simulink model "DCM_17_Parrllel_Pairs_18Ms"  (R2019b)
settings: Solver=VariableStepAuto  StartTime=0.0  StopTime=20  RelTol=1e-3
model workspace (MAT data in the model file):
  Laf = 0.00735
  Laf_2 = 0.00844
  Rarm = 0.0096
  angular_vel = 145
  angular_vel_1 = 175.405
  angular_vel_10 = 168.703
  angular_vel_11 = 168.598
  angular_vel_12 = 167.865
  angular_vel_13 = 167.132
  angular_vel_14 = 166.923
  angular_vel_15 = 165.666
  angular_vel_16 = 164.41
  angular_vel_2 = 173.625
  angular_vel_3 = 172.787
  angular_vel_4 = 170.902
  angular_vel_5 = 170.902
  angular_vel_6 = 169.96
  angular_vel_7 = 169.855
  angular_vel_8 = 169.122
libraries: powerlib x74, simulink x1
settings Model: OrderedModelArguments=off  Creator=Sy2  LastModifiedBy=Sy2
settings SolverCC: ZeroCrossAlgorithm=Adaptive
settings DebuggingCC: IgnoredZcDiagnostic=none

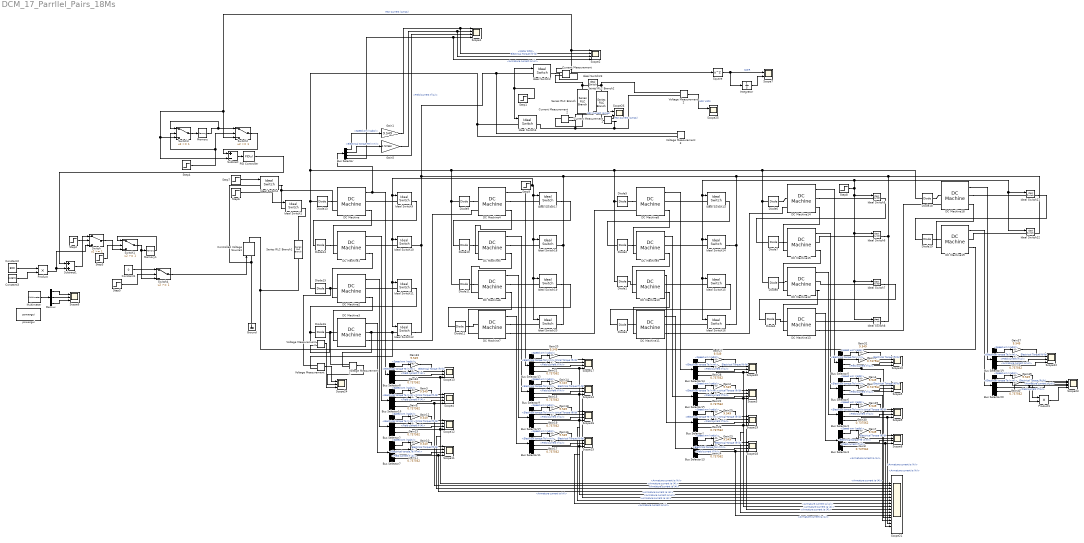
== system DCM_17_Parrllel_Pairs_18Ms ==
  Bus Selector{,1..16,19..20} (19 alike) : BusSelector  OutputSignals=Speed wm (rad/s),Electrical torque Te (n m),Field current if (A),Armature current ia (A)
  Constant1 : Constant  Value=0
  Constant2 : Constant  Value=800
  Constant3 : Constant  Value=0.0972
  Controlled Voltage Source1 : powerlib/Electrical Sources/Controlled Voltage Source  Initialize=on  Source_Type=DC  Amplitude=0  Phase=0  Frequency=0  Measurements=Voltage
      settings: SourceProductName=Simscape Electrical
  Current Measurement : powerlib/Measurements/Current Measurement  PhasorSimulation=off  OutputType=Complex  PSBequivalent=0
      settings: SourceProductName=Simscape Electrical
  Current Measurement1 : powerlib/Measurements/Current Measurement  PhasorSimulation=off  OutputType=Complex  PSBequivalent=0
      settings: SourceProductName=Simscape Electrical
  Current Measurement2 : powerlib/Measurements/Current Measurement  PhasorSimulation=off  OutputType=Complex  PSBequivalent=0
      settings: SourceProductName=Simscape Electrical
  DC Machine{,1..15,18..19} (18 alike) : powerlib/Machines/DC Machine  PresetModel=No  MechanicalLoad=Torque TL  FieldType=Wound  ShowDetailedParameters=on  MeasurementBus=off  RLa="[Rarm  0.002]"  RLf=[0.0054 0.0125]  Laf=Laf  MachineConstant=Torque constant (N.m/A)  Ke=1.8  Kt=1.8  J=137  Bm=0  Tf=0  w0=angular_vel  Ifinit=0  TsPowergui=0  TsBlock=-1
      settings: SourceProductName=Simscape Electrical
  Demux : Demux  Outputs=3
  Diode{1..2,4,6..12,14,18..19} (13 alike) : powerlib/Power Electronics/Diode  Ron=0.001  Lon=0  Vf=0.8  IC=0  UseSnubber=0  Rs=500000  Cs=250e-9  Measurements=off
      settings: SourceProductName=Simscape Electrical
  Diode13 : powerlib/Power Electronics/Diode  Ron=0.0000001  Lon=0  Vf=0.8  IC=0  UseSnubber=0  Rs=500000  Cs=250e-9  Measurements=off
      settings: SourceProductName=Simscape Electrical
  Diode15 : powerlib/Power Electronics/Diode  Ron=0.000000000001  Lon=0  Vf=0.8  IC=0  UseSnubber=0  Rs=inf  Cs=0  Measurements=off
      settings: SourceProductName=Simscape Electrical
  Diode16 : powerlib/Power Electronics/Diode  Ron=0.000000001  Lon=0  Vf=0.8  IC=0  UseSnubber=0  Rs=inf  Cs=0  Measurements=off
      settings: SourceProductName=Simscape Electrical
  Diode3 : powerlib/Power Electronics/Diode  Ron=0.00001  Lon=0  Vf=0.8  IC=0  UseSnubber=0  Rs=500000  Cs=250e-9  Measurements=off
      settings: SourceProductName=Simscape Electrical
  Diode5 : powerlib/Power Electronics/Diode  Ron=0.000001  Lon=0  Vf=0.8  IC=0  UseSnubber=0  Rs=500000  Cs=250e-9  Measurements=off
      settings: SourceProductName=Simscape Electrical
  Gain{1..4,7,10,12,14,16,18,20,23,25,27,29,31,33,37,39} (19 alike) : Gain  Gain=9.549
  Gain{5..6,8..9,11,13,15,17,19,21..22,24,26,28,30,32,34,38,40} (19 alike) : Gain  Gain=0.737562
  Ground : powerlib/Elements/Ground  LConnTagsString=a
      settings: SourceProductName=Simscape Electrical
  Ideal Switch{1..3,5..23} (22 alike) : powerlib/Power Electronics/Ideal Switch  Ron=0  Lon=0  IC=0  Rs=inf  Cs=0  Measurements=on
      settings: SourceProductName=Simscape Electrical
  Ideal Switch4 : powerlib/Power Electronics/Ideal Switch  Ron=0  Lon=0  IC=1  Rs=inf  Cs=0  Measurements=on
      settings: SourceProductName=Simscape Electrical
  Integrator : Integrator  ZeroCross=off
  Memory : Memory
  Memory1 : Memory
  Multimeter : powerlib/Measurements/Multimeter  PhasorSimulation=off  OutputType=Complex  sel=[2 3 1]  L=3  Gain=[1 1 1]  yselected={'Usrc: Controlled Voltage Source1','Ib: Series RLC Branch1','Ub: Series RLC Branch1'};  PSBOutputType=1  PSBequivalent=0  AxesSetting=[0,0.1,-100,100]  Display=0  SavedBlockNames=-11
      settings: SourceProductName=Simscape Electrical
  PID Controller : simulink/Continuous/PID Controller  Controller=PID  Form=Parallel  TimeDomain=Continuous-time  SampleTime=-1  IntegratorMethod=Forward Euler  FilterMethod=Forward Euler  ControllerParametersSource=internal  P=10  I=7  D=1  UseFilter=on  N=100  TunerSelectOption=Transfer Function Based (PID Tuner App)  InitialConditionSource=internal  InitialConditionForIntegrator=0  InitialConditionForFilter=0  DifferentiatorICPrevScaledInput=0  ExternalReset=none  TrackingMode=off  Kt=1  LimitOutput=off  UpperSaturationLimit=inf  LowerSaturationLimit=-inf  LinearizeAsGain=on  AntiWindupMode=none  Kb=1  POutMin=[]  POutMax=[]  IOutMin=[]  IOutMax=[]  DOutMin=[]  DOutMax=[]  NOutMin=[]  NOutMax=[]  SumOutMin=[]  SumOutMax=[]  SaturationOutMin=[]  SaturationOutMax=[]  PParamMin=[]  PParamMax=[]  IParamMin=[]  IParamMax=[]  DParamMin=[]  DParamMax=[]  NParamMin=[]  NParamMax=[]  KbParamMin=[]  KbParamMax=[]  KtParamMin=[]  KtParamMax=[]  KbOutMin=[]  KbOutMax=[]  KtOutMin=[]  KtOutMax=[]  IntegratorOutMin=[]  IntegratorOutMax=[]  FilterOutMin=[]  FilterOutMax=[]  SumI1OutMin=[]  SumI1OutMax=[]  SumI2OutMin=[]  SumI2OutMax=[]  SumI3OutMin=[]  SumI3OutMax=[]  SumI4OutMin=[]  SumI4OutMax=[]  SumDOutMin=[]  SumDOutMax=[]  DifferentiatorOutMin=[]  DifferentiatorOutMax=[]  FilterDiffOutCoefMin=[]  FilterDiffOutCoefMax=[]  ReciprocalOutMin=[]  ReciprocalOutMax=[]  SumDenOutMin=[]  SumDenOutMax=[]  SumNumOutMin=[]  SumNumOutMax=[]  DivideOutMin=[]  DivideOutMax=[]  IntegratorContinuousStateAttributes=''  IntegratorStateMustResolveToSignalObject=off  IntegratorRTWStateStorageClass=Auto  FilterContinuousStateAttributes=''  FilterStateMustResolveToSignalObject=off  FilterRTWStateStorageClass=Auto  ParallelPVariant=InternalParameters  IdealPVariant=Disabled  IVariant=InternalParameters  DVariant=InternalParameters  IntegratorVariant=Continuous  SatVariant=Disabled  AWVariant=Passthrough  PCopyVariant=Disabled  TRVariant=Disabled  FdbkBlocksVariant=Forward  IdealPFdbkVariant=Disabled  SatFdbkVariant=Disabled  DerivativeFilterVariant=ContFilter  NVariant=InternalParameters  NCopyVariant=Disabled  FilterICVariant=InternalICsFilter  IntegratorICVariant=InternalICs  ExternalResetVariant=Disabled  TRSumVariant=Passthrough  SumFdbkVariant=Disabled  SumVariant=Sum_PID
  Product : Product
  Product1 : Product
  Scope{1..5,8..20,22} (19 alike) : Scope  NumInputPorts=4
  Scope21 : Scope  NumInputPorts=16
  Scope23 : Scope  NumInputPorts=5
  Scope24 : Scope  NumInputPorts=3
  Scope25 : Scope  NumInputPorts=2
  Scope26 : Scope  NumInputPorts=2
  Scope6 : Scope  NumInputPorts=3
  Scope7 : Scope  NumInputPorts=2
  Series RLC Branch : powerlib/Elements/Series RLC Branch  LConnTagsString=__new0  RConnTagsString=__new0  BranchType=RL  Resistance=0.09  Inductance=0.02  SetiL0=off  InitialCurrent=0  Capacitance=1e-6  Setx0=off  InitialVoltage=0  Measurements=None
      settings: SourceProductName=Simscape Electrical
  Series RLC Branch1 : powerlib/Elements/Series RLC Branch  Description=Field Dump Resistor  LConnTagsString=__new0  RConnTagsString=__new0  BranchType=R  Resistance=5  Inductance=1e-3  SetiL0=off  InitialCurrent=0  Capacitance=1e-6  Setx0=off  InitialVoltage=0  Measurements=Branch voltage and current
      settings: AttributesFormatString=%<Description>  SourceProductName=Simscape Electrical
  Series RLC Branch2 : powerlib/Elements/Series RLC Branch  LConnTagsString=__new0  RConnTagsString=__new0  BranchType=RL  Resistance=0.90  Inductance=0.015  SetiL0=off  InitialCurrent=0  Capacitance=1e-6  Setx0=off  InitialVoltage=0  Measurements=None
      settings: SourceProductName=Simscape Electrical
  Square : Math  Operator=square  RndMeth=Zero  SaturateOnIntegerOverflow=on
  Step1 : Step  Time=12  SampleTime=0  VectorParams1D=off
  Step{2..3,5..6} (4 alike) : Step  Time=13  SampleTime=0  VectorParams1D=off  ZeroCross=off
  Step4 : Step  Time=12.72  SampleTime=0  VectorParams1D=off  ZeroCross=off
  Step7 : Step  Time=13  Before=1  After=0  SampleTime=0  VectorParams1D=off  ZeroCross=off
  Step8 : Step  Time=12  SampleTime=0  VectorParams1D=off
  Step9 : Step  Time=12  SampleTime=0  VectorParams1D=off
  Subtract : Sum  Inputs=+-
  Subtract1 : Sum
  Switch{,1..4} (5 alike) : Switch  Threshold=1  ZeroCross=off
  Voltage Measurement{,1..4} (5 alike) : powerlib/Measurements/Voltage Measurement  PhasorSimulation=off  OutputType=Complex  PSBequivalent=0
      settings: SourceProductName=Simscape Electrical
  powergui : powerlib/powergui  Priority=1  SimulationMode=Continuous  SampleTime=50e-6  frequency=60  Iterations=50  frequencyindice=0  Pbase=100e6  ErrMax=1e-4  UnitsV=kV  UnitsW=MW  buscounter=0  FunctionMessages=off  echomessages=off  EnableUseOfTLC=off  CurrentSourceSwitches=off  DisableSnubberDevices=off  DisableRonSwitches=off  DisableVfSwitches=off  DisplayEquations=off  AutomaticDiscreteSolvers=off  SolverType=Tustin/Backward Euler (TBE)  Interpol=off  ExternalGateDelay=off  methode=off  Ts=100  x0status=blocks  SPID=on  SwTol=0  HookPort=off  NonlinearTolerance=1e-4  nMaxIteration=100  ContinueOnMaxIteration=off  RestoreLinks=warning  ResistiveCurrentMeasurement=off  Frange=[0:2:500]  Ylog=off  Xlog=on  ShowGrid=off  save=off  variable=ZData  structure=0  ZoomFFT=off  StartTime=0.0  cycles=1  DisplayStyle=1  fundamental=60  FreqAxis=off  MaxFrequency=1000  frequencyindicesteady=1  RmsSteady=1  display=off
      settings: SourceProductName=Simscape Electrical
  wires:
  Bus Selector/1 -> Gain1/1  "<Speed wm (rad/s)>"
  Bus Selector/3 -> Scope1/3  "<Field current if (A)>"
  Bus Selector/4 -> Scope2/4, Scope1/4  "<Armature current ia (A)>"
  Gain1/1 -> Scope1/1, Scope2/2  "<Motor RPM>"
  Step1/1 -> Ideal Switch2/1, Ideal Switch3/1
  Step2/1 -> Switch/2
  Current Measurement/1 -> Square/1, Switch2/3, Switch3/3, Subtract/2, Scope2/1  "HSX Current (Amps)"
  Memory/1 -> Switch3/1, Switch2/1
  Subtract/1 -> PID Controller/1
  PID Controller/1 -> Subtract1/1
  Constant2/1 -> Product/1
  Subtract1/1 -> Switch/1
  Step3/1 -> Switch1/2
  Switch2/1 -> Subtract/1
  Step4/1 -> Switch2/2, Switch3/2
  Switch3/1 -> Memory/1
  Bus Selector/2 -> Gain5/1  "<Electrical torque Te (n m)>"
  Gain5/1 -> Scope2/3, Scope1/2  "Electrical Torque (ft-lb)"
  Square/1 -> Scope7/1, Integrator/1  "Isq*R"
  Integrator/1 -> Scope7/2
  Switch4/1 -> Controlled Voltage Source1/1
  Step5/1 -> Switch4/2
  Constant1/1 -> Switch4/1
  Step6/1 -> Ideal Switch1/1
  Step7/1 -> Ideal Switch4/1
  Constant3/1 -> Product/2
  Product/1 -> Subtract1/2, Switch/3
  Switch/1 -> Switch1/3
  Switch1/1 -> Switch4/3, Memory1/1
  Memory1/1 -> Switch1/1
  Demux/2 -> Scope6/2
  Multimeter/1 -> Demux/1
  Demux/1 -> Scope6/1
  Demux/3 -> Scope6/3
  Step9/1 -> Ideal Switch12/1, Ideal Switch11/1, Ideal Switch10/1, Ideal Switch9/1, Ideal Switch17/1, Ideal Switch19/1, Ideal Switch20/1, Ideal Switch18/1
  Bus Selector9/2 -> Gain15/1  "<Electrical torque Te (n m)>"
  Bus Selector9/3 -> Scope14/3  "<Field current if (A)>"
  DC Machine5/1 -> Bus Selector9/1
  Bus Selector10/3 -> Scope16/3  "<Field current if (A)>"
  Gain15/1 -> Scope14/2  "Electrical Torque (ft-lb)"
  Bus Selector9/4 -> Scope21/6, Scope14/4  "<Armature current ia (A)>"
  Gain14/1 -> Scope14/1
  Bus Selector9/1 -> Gain14/1  "<Speed wm (rad/s)>"
  Bus Selector10/1 -> Gain18/1  "<Speed wm (rad/s)>"
  DC Machine7/1 -> Bus Selector11/1
  Gain19/1 -> Scope16/2  "Electrical Torque (ft-lb)"
  Bus Selector11/4 -> Scope21/8, Scope15/4  "<Armature current ia (A)>"
  Bus Selector10/4 -> Scope21/7, Scope16/4  "<Armature current ia (A)>"
  Gain18/1 -> Scope16/1
  DC Machine6/1 -> Bus Selector10/1
  Gain16/1 -> Scope15/1
  Bus Selector11/1 -> Gain16/1  "<Speed wm (rad/s)>"
  Bus Selector11/3 -> Scope15/3  "<Field current if (A)>"
  Bus Selector11/2 -> Gain17/1  "<Electrical torque Te (n m)>"
  Gain17/1 -> Scope15/2  "Electrical Torque (ft-lb)"
  Bus Selector10/2 -> Gain19/1  "<Electrical torque Te (n m)>"
  Gain20/1 -> Scope17/1
  Bus Selector12/4 -> Scope21/5, Scope17/4  "<Armature current ia (A)>"
  Gain21/1 -> Scope17/2  "Electrical Torque (ft-lb)"
  Bus Selector12/1 -> Gain20/1  "<Speed wm (rad/s)>"
  Bus Selector12/3 -> Scope17/3  "<Field current if (A)>"
  Bus Selector12/2 -> Gain21/1  "<Electrical torque Te (n m)>"
  DC Machine4/1 -> Bus Selector12/1
  DC Machine10/1 -> Bus Selector1/1
  Bus Selector14/3 -> Scope20/3  "<Field current if (A)>"
  Bus Selector14/2 -> Gain28/1  "<Electrical torque Te (n m)>"
  Gain28/1 -> Scope20/2  "Electrical Torque (ft-lb)"
  Bus Selector14/1 -> Gain27/1  "<Speed wm (rad/s)>"
  Gain27/1 -> Scope20/1
  Bus Selector14/4 -> Scope21/9, Scope20/4  "<Armature current ia (A)>"
  DC Machine8/1 -> Bus Selector14/1
  Bus Selector13/1 -> Gain23/1  "<Speed wm (rad/s)>"
  Gain24/1 -> Scope18/2  "Electrical Torque (ft-lb)"
  Gain23/1 -> Scope18/1
  Bus Selector13/2 -> Gain24/1  "<Electrical torque Te (n m)>"
  Gain25/1 -> Scope19/1
  DC Machine9/1 -> Bus Selector15/1
  Gain26/1 -> Scope19/2  "Electrical Torque (ft-lb)"
  Bus Selector13/3 -> Scope18/3  "<Field current if (A)>"
  Bus Selector1/1 -> Gain25/1  "<Speed wm (rad/s)>"
  Gain2/1 -> Scope3/1
  Bus Selector1/3 -> Scope19/3  "<Field current if (A)>"
  Bus Selector1/4 -> Scope21/11, Scope19/4  "<Armature current ia (A)>"
  Bus Selector15/4 -> Scope21/10, Scope3/4  "<Armature current ia (A)>"
  Gain22/1 -> Scope3/2  "Electrical Torque (ft-lb)"
  DC Machine11/1 -> Bus Selector13/1
  Bus Selector15/1 -> Gain2/1  "<Speed wm (rad/s)>"
  Bus Selector1/2 -> Gain26/1  "<Electrical torque Te (n m)>"
  Bus Selector15/3 -> Scope3/3  "<Field current if (A)>"
  Bus Selector15/2 -> Gain22/1  "<Electrical torque Te (n m)>"
  DC Machine12/1 -> Bus Selector3/1
  Bus Selector5/3 -> Scope10/3  "<Field current if (A)>"
  Bus Selector5/2 -> Gain32/1  "<Electrical torque Te (n m)>"
  Gain32/1 -> Scope10/2  "Electrical Torque (ft-lb)"
  Bus Selector5/1 -> Gain31/1  "<Speed wm (rad/s)>"
  Gain31/1 -> Scope10/1
  Bus Selector5/4 -> Scope21/13, Scope10/4  "<Armature current ia (A)>"
  DC Machine14/1 -> Bus Selector5/1
  Bus Selector4/1 -> Gain7/1  "<Speed wm (rad/s)>"
  Gain8/1 -> Scope8/2  "Electrical Torque (ft-lb)"
  Gain7/1 -> Scope8/1
  Bus Selector4/2 -> Gain8/1  "<Electrical torque Te (n m)>"
  Gain29/1 -> Scope9/1
  DC Machine15/1 -> Bus Selector6/1
  Gain30/1 -> Scope9/2  "Electrical Torque (ft-lb)"
  Bus Selector4/3 -> Scope8/3  "<Field current if (A)>"
  Bus Selector4/4 -> Scope8/4, Scope21/16  "<Armature current ia (A)>"
  Bus Selector3/1 -> Gain29/1  "<Speed wm (rad/s)>"
  Gain4/1 -> Scope5/1
  Bus Selector3/3 -> Scope9/3  "<Field current if (A)>"
  Bus Selector3/4 -> Scope21/15, Scope9/4  "<Armature current ia (A)>"
  Bus Selector6/4 -> Scope21/14, Scope5/4  "<Armature current ia (A)>"
  Gain6/1 -> Scope5/2  "Electrical Torque (ft-lb)"
  DC Machine13/1 -> Bus Selector4/1
  Bus Selector6/1 -> Gain4/1  "<Speed wm (rad/s)>"
  Bus Selector3/2 -> Gain30/1  "<Electrical torque Te (n m)>"
  Bus Selector6/3 -> Scope5/3  "<Field current if (A)>"
  Bus Selector6/2 -> Gain6/1  "<Electrical torque Te (n m)>"
  DC Machine2/1 -> Bus Selector2/1
  Bus Selector8/3 -> Scope13/3  "<Field current if (A)>"
  Bus Selector8/2 -> Gain34/1  "<Electrical torque Te (n m)>"
  Gain34/1 -> Scope13/2  "Electrical Torque (ft-lb)"
  Bus Selector8/1 -> Gain33/1  "<Speed wm (rad/s)>"
  Gain33/1 -> Scope13/1
  Bus Selector8/4 -> Scope21/1, Scope13/4  "<Armature current ia (A)>"
  DC Machine/1 -> Bus Selector8/1, Bus Selector/1
  Bus Selector7/1 -> Gain10/1  "<Speed wm (rad/s)>"
  Gain11/1 -> Scope11/2  "Electrical Torque (ft-lb)"
  Gain10/1 -> Scope11/1
  Bus Selector7/2 -> Gain11/1  "<Electrical torque Te (n m)>"
  Gain12/1 -> Scope12/1
  DC Machine1/1 -> Bus Selector16/1
  Gain13/1 -> Scope12/2  "Electrical Torque (ft-lb)"
  Bus Selector7/3 -> Scope11/3  "<Field current if (A)>"
  Bus Selector7/4 -> Scope11/4, Scope21/4  "<Armature current ia (A)>"
  Bus Selector2/1 -> Gain12/1  "<Speed wm (rad/s)>"
  Gain3/1 -> Scope4/1
  Bus Selector2/3 -> Scope12/3  "<Field current if (A)>"
  Bus Selector2/4 -> Scope21/3, Scope12/4  "<Armature current ia (A)>"
  Gain9/1 -> Scope4/2  "Electrical Torque (ft-lb)"
  DC Machine3/1 -> Bus Selector7/1
  Bus Selector16/1 -> Gain3/1  "<Speed wm (rad/s)>"
  Bus Selector2/2 -> Gain13/1  "<Electrical torque Te (n m)>"
  Bus Selector16/3 -> Scope4/3  "<Field current if (A)>"
  Bus Selector16/2 -> Gain9/1  "<Electrical torque Te (n m)>"
  Bus Selector16/4 -> Scope21/2, Scope4/4  "<Armature current ia (A)>"
  Bus Selector13/4 -> Scope21/12, Scope18/4  "<Armature current ia (A)>"
  Bus Selector19/3 -> Scope22/3  "<Field current if (A)>"
  Gain40/1 -> Scope23/2  "Electrical Torque (ft-lb)"
  Bus Selector20/1 -> Gain39/1  "<Speed wm (rad/s)>"
  Bus Selector19/1 -> Gain37/1  "<Speed wm (rad/s)>"
  Bus Selector20/3 -> Scope23/3  "<Field current if (A)>"
  Bus Selector19/2 -> Gain38/1  "<Electrical torque Te (n m)>"
  Bus Selector19/4 -> Scope22/4  "<Armature current ia (A)>"
  DC Machine18/1 -> Bus Selector19/1
  Gain37/1 -> Scope22/1
  Step8/1 -> Ideal Switch22/1, Ideal Switch21/1, Ideal Switch15/1, Ideal Switch16/1, Ideal Switch14/1, Ideal Switch13/1, Ideal Switch8/1, Ideal Switch7/1, Ideal Switch6/1, Ideal Switch5/1
  DC Machine19/1 -> Bus Selector20/1
  Bus Selector20/4 -> Product1/2, Scope23/4  "<Armature current ia (A)>"
  Gain38/1 -> Scope22/2  "Electrical Torque (ft-lb)"
  Bus Selector20/2 -> Gain40/1  "<Electrical torque Te (n m)>"
  Gain39/1 -> Product1/1, Scope23/1
  Voltage Measurement/1 -> Scope24/1
  Voltage Measurement1/1 -> Scope24/2
  Voltage Measurement2/1 -> Scope25/1  "HSX Volts"
  Voltage Measurement4/1 -> Scope24/3
  Current Measurement2/1 -> Scope26/1  "HSX Current (Amps)"
  Current Measurement1/1 -> Scope26/2  "HSX Current (Amps)"
  Product1/1 -> Scope23/5
  connections:
  Voltage Measurement2/LConn2 -- Current Measurement1/RConn1 -- Ideal Switch3/RConn1 -- Current Measurement2/RConn1
  Ideal Switch12/RConn1 -- Ideal Switch20/RConn1 -- Ideal Switch18/RConn1 -- Ideal Switch8/RConn1 -- Ideal Switch6/RConn1 -- Ideal Switch22/RConn1 -- Ideal Switch16/RConn1 -- Ideal Switch14/RConn1 -- Ideal Switch2/LConn1 -- Voltage Measurement3/LConn1 -- Ideal Switch10/RConn1
  DC Machine/RConn2 -- DC Machine1/LConn2
  DC Machine1/RConn2 -- DC Machine2/LConn2
  DC Machine2/RConn2 -- DC Machine3/LConn2
  DC Machine3/RConn2 -- DC Machine4/LConn2
  DC Machine4/RConn2 -- DC Machine5/LConn2
  DC Machine5/RConn2 -- DC Machine6/LConn2
  DC Machine6/RConn2 -- DC Machine7/LConn2
  DC Machine7/RConn2 -- DC Machine8/LConn2
  DC Machine8/RConn2 -- DC Machine9/LConn2
  DC Machine9/RConn2 -- DC Machine10/LConn2
  DC Machine10/RConn2 -- DC Machine11/LConn2
  DC Machine11/RConn2 -- DC Machine14/LConn2
  DC Machine14/RConn2 -- DC Machine15/LConn2
  DC Machine15/RConn2 -- DC Machine12/LConn2
  DC Machine12/RConn2 -- DC Machine13/LConn2
  DC Machine/LConn2 -- Ideal Switch4/RConn1 -- Ideal Switch1/LConn1
  Ideal Switch1/RConn1 -- Series RLC Branch1/LConn1
  Ideal Switch9/LConn1 -- DC Machine/RConn1
  Ideal Switch10/LConn1 -- DC Machine1/RConn1
  Ideal Switch11/LConn1 -- DC Machine2/RConn1
  DC Machine3/RConn1 -- Voltage Measurement1/LConn2 -- Voltage Measurement/LConn2 -- Ideal Switch12/LConn1
  Ideal Switch13/LConn1 -- DC Machine8/RConn1
  Ideal Switch14/LConn1 -- DC Machine9/RConn1
  Ideal Switch15/LConn1 -- DC Machine10/RConn1
  Ideal Switch16/LConn1 -- DC Machine11/RConn1
  DC Machine7/RConn1 -- Ideal Switch20/LConn1
  DC Machine6/RConn1 -- Ideal Switch19/LConn1
  DC Machine5/RConn1 -- Ideal Switch18/LConn1
  DC Machine4/RConn1 -- Ideal Switch17/LConn1
  Diode14/RConn1 -- DC Machine1/LConn1
  Diode13/RConn1 -- DC Machine/LConn1
  DC Machine14/RConn1 -- Ideal Switch5/LConn1
  Diode8/RConn1 -- DC Machine12/LConn1
  Diode4/RConn1 -- DC Machine13/LConn1
  Ideal Switch6/LConn1 -- DC Machine15/RConn1
  Ideal Switch7/LConn1 -- DC Machine12/RConn1
  Ideal Switch8/LConn1 -- DC Machine13/RConn1
  Diode2/RConn1 -- DC Machine9/LConn1
  DC Machine10/LConn1 -- Diode1/RConn1
  DC Machine11/LConn1 -- Diode3/RConn1
  Diode5/RConn1 -- DC Machine8/LConn1
  Diode15/RConn1 -- Voltage Measurement/LConn1 -- DC Machine2/LConn1
  Diode16/RConn1 -- DC Machine3/LConn1 -- Voltage Measurement4/LConn2 -- Voltage Measurement1/LConn1
  Diode9/RConn1 -- DC Machine4/LConn1
  Diode10/RConn1 -- DC Machine5/LConn1
  Diode11/RConn1 -- DC Machine6/LConn1
  Diode12/RConn1 -- DC Machine7/LConn1
  Diode6/RConn1 -- DC Machine14/LConn1
  Diode7/RConn1 -- DC Machine15/LConn1
  Ground/LConn1 -- Controlled Voltage Source1/LConn1 -- Ideal Switch4/LConn1
  Series RLC Branch2/LConn1 -- Ideal Switch23/RConn1 -- Voltage Measurement2/LConn1
  Controlled Voltage Source1/RConn1 -- DC Machine19/RConn2 -- Series RLC Branch1/RConn1
  DC Machine18/RConn2 -- DC Machine19/LConn2
  DC Machine18/RConn1 -- Ideal Switch21/LConn1
  Ideal Switch22/LConn1 -- DC Machine19/RConn1
  Diode19/RConn1 -- DC Machine19/LConn1
  Diode18/RConn1 -- DC Machine18/LConn1
  DC Machine13/RConn2 -- DC Machine18/LConn2
  Ideal Switch9/RConn1 -- Diode14/LConn1
  Ideal Switch11/RConn1 -- Voltage Measurement4/LConn1 -- Diode16/LConn1
  Ideal Switch17/RConn1 -- Diode10/LConn1
  Ideal Switch19/RConn1 -- Diode12/LConn1
  Diode2/LConn1 -- Ideal Switch13/RConn1
  Ideal Switch15/RConn1 -- Diode3/LConn1
  Diode7/LConn1 -- Ideal Switch5/RConn1
  Ideal Switch7/RConn1 -- Diode4/LConn1
  Ideal Switch21/RConn1 -- Diode19/LConn1
  Diode18/LConn1 -- Diode1/LConn1 -- Diode5/LConn1 -- Diode11/LConn1 -- Diode9/LConn1 -- Voltage Measurement3/LConn2 -- Ideal Switch3/LConn1 -- Diode15/LConn1 -- Diode13/LConn1 -- Diode8/LConn1 -- Diode6/LConn1
  Ideal Switch2/RConn1 -- Current Measurement/LConn1
  Series RLC Branch/RConn1 -- Current Measurement2/LConn1
  Series RLC Branch2/RConn1 -- Current Measurement1/LConn1
  Current Measurement/RConn1 -- Ideal Switch23/LConn1 -- Series RLC Branch/LConn1
